simulink library "powerlib_models"  (Simulink 6.0)
settings: Solver=ode45  SolverMode=SingleTasking  StartTime=0.0  StopTime=10.0  RelTol=1e-3
values from neighbouring files (symbols this model uses):
  Ts = get(handles.edit1,'string')    [powergui.m]
undefined symbols (not defined in the file or in its folder): A, a0, a1, a2, a3, a4, a5, Ac, Amplitude, Amplitudes, B, BaseCurrent, BaseFlux, Bc, C, Capacitance, Cc, Columns, ConnectionType, Cs, ctrl, current, Current, damp, Dc, Dd, DiscIntNeverNeededParam, dref, dwo, exc, excAxis, F, Flux, fnom, Frequency, FreqVps, Gain1, gate, GH, GHd, GI, GId, GL, GLd, H, HarmonicGeneration, HT, hyd, I1_init, ib, ib2, Id1o, Inductance, InitialFlux, InitialSlope, io, Iq1o, isfinite, j, J ... (+138)
libraries: powerlib_models x32, powerlib_extras x4
(part 2 of 11)

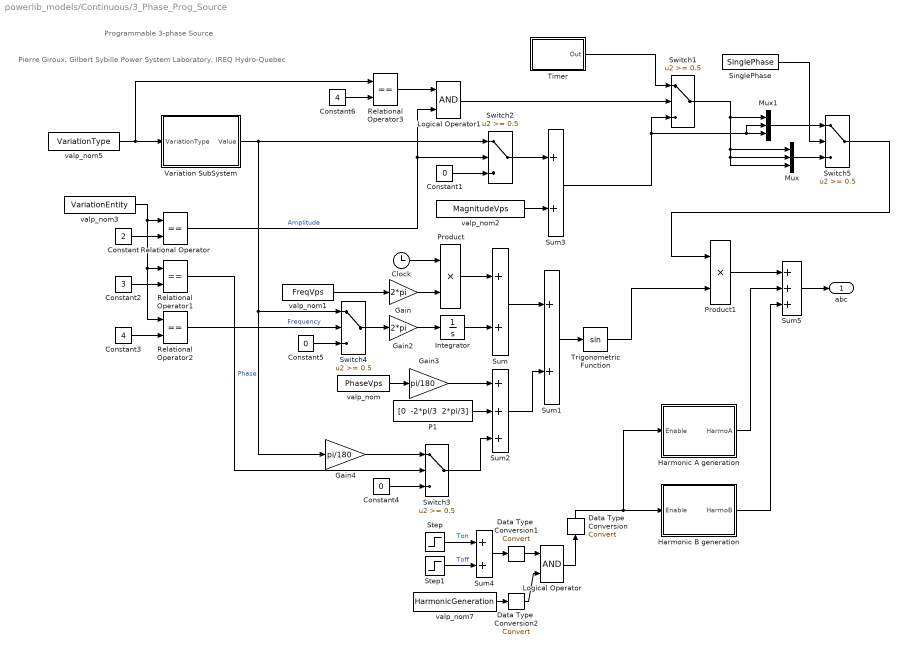
== system powerlib_models/Continuous/3_Phase_Prog_Source ==
  note: Pierre Giroux, Gilbert Sybille
      | Power System Laboratory, IREQ
      | Hydro-Quebec
  note: Programmable 3-phase Source
  Clock : Clock
  Constant : Constant  Value=2
  Constant1 : Constant  Value=0
  Constant2 : Constant  Value=3
  Constant3 : Constant  Value=4
  Constant4 : Constant  Value=0
  Constant5 : Constant  Value=0
  Constant6 : Constant  Value=4
  Data Type  Conversion : DataTypeConversion  Orientation=up  OutDataTypeMode=double  SaturateOnIntegerOverflow=on  RndMeth=Zero
  Data Type  Conversion1 : DataTypeConversion  OutDataTypeMode=boolean  SaturateOnIntegerOverflow=on  RndMeth=Zero
  Data Type  Conversion2 : DataTypeConversion  OutDataTypeMode=boolean  SaturateOnIntegerOverflow=on  RndMeth=Zero
  Gain : Gain  Gain=2*pi  SaturateOnIntegerOverflow=on
  Gain2 : Gain  Gain=2*pi  SaturateOnIntegerOverflow=on
  Gain3 : Gain  Gain=pi/180  SaturateOnIntegerOverflow=on
  Gain4 : Gain  Gain=pi/180  SaturateOnIntegerOverflow=on
  Harmonic A generation : Subsystem  mask(Harmonic generation){Freq_Vps=FreqVps, n_Harmo=n_HarmoA, Mag_Harmo=Mag_HarmoA, Phase_Harmo=Phase_HarmoA, Seq_Harmo=Seq_HarmoA, Ts=0}
      mask prompts: Ts "Sample time:"
  Harmonic B generation : Subsystem  mask(Harmonic generation){Freq_Vps=FreqVps, n_Harmo=n_HarmoB, Mag_Harmo=Mag_HarmoB, Phase_Harmo=Phase_HarmoB, Seq_Harmo=Seq_HarmoB, Ts=0}
      mask prompts: Ts "Sample time:"
  Integrator : Integrator
  Logical Operator : Logic
  Logical Operator1 : Logic
  Mux : Mux  Inputs=3
  Mux1 : Mux  Inputs=3
  P1 : Constant  Value="[0  -2*pi/3  2*pi/3]"
  Product : Product  SaturateOnIntegerOverflow=on  InputSameDT=on
  Product1 : Product  SaturateOnIntegerOverflow=on  InputSameDT=on
  Relational Operator{,1..3} (4 alike) : RelationalOperator  Operator===  InputSameDT=on
  SinglePhase : Constant  Value=SinglePhase
  Step : Step  Time=Ton_Harmo  SampleTime=0
  Step1 : Step  Time=Toff_Harmo  After=-1  SampleTime=0
  Sum{,1,3..4} (4 alike) : Sum  SaturateOnIntegerOverflow=on  InputSameDT=on
  Sum2 : Sum  Inputs=+++  SaturateOnIntegerOverflow=on  InputSameDT=on
  Sum5 : Sum  Inputs=+++  SaturateOnIntegerOverflow=on  InputSameDT=on
  Switch{1..5} (5 alike) : Switch  Threshold=0.5  InputSameDT=on
  Timer : Subsystem  mask(Timer){t=TimeValues, e=Amplitudes, Ts=0}
      mask prompts: t "Time (s):"; e "Amplitude:"; Ts "Sample time (s)"
      mask help:
      | Generates a signal changing  at specified times.
      |
      | Value of the signal at time zero must  be specified.
      mask init:
      | tt=t;sv=e;
      | tv=[-1,tt(1),reshape(repmat(reshape(tt(2:end),1,length(tt)-1),2,1),1,2*length(tt)-2),tt(end)+1];
      | %sv=(sv(:)'~=0);
      | opv=[sv(1),reshape(repmat(sv(1:end-1),2,1),1,2*length(sv)-2),sv(end),sv(end)];
      mask Display: plot( tv(2:end-1), opv(2:end-1) )
  Trigonometric Function : Trigonometry
  Variation SubSystem : Subsystem  mask(Variation Subsystem){VariationStep=VariationStep, VariationRate=VariationRate, VariationFreq=VariationFrequency, VariationMag=VariationMagnitude, Ton_Variation=Ton_Variation, Toff_Variation=Toff_Variation, Ts=0}
      mask prompts: Ts "Sample time:"
  valp_nom : Constant  Value=PhaseVps
  valp_nom1 : Constant  Value=FreqVps
  valp_nom2 : Constant  Value=MagnitudeVps
  valp_nom3 : Constant  Value=VariationEntity
  valp_nom5 : Constant  Value=VariationType
  valp_nom7 : Constant  Value=HarmonicGeneration
  abc : Outport  InitialOutput=0
  wires:
  Logical Operator1/1 -> Switch1/2
  Relational Operator3/1 -> Logical Operator1/1
  Switch5/1 -> Product1/1
  Switch1/1 -> Mux1/1, Mux/3, Mux/2, Mux/1
  Mux/1 -> Switch5/3
  SinglePhase/1 -> Switch5/2
  Mux1/1 -> Switch5/1
  Timer/1(Out) -> Switch1/1
  Sum3/1 -> Mux1/2, Mux1/3, Switch1/3
  Constant6/1 -> Relational Operator3/2
  Gain4/1 -> Switch3/1
  Harmonic B generation/1(HarmoB) -> Sum5/3
  Step1/1 -> Sum4/2  "Toff"
  Step/1 -> Sum4/1  "Ton"
  Sum5/1 -> abc/1
  Harmonic A generation/1(HarmoA) -> Sum5/2
  Constant5/1 -> Switch4/3
  Constant3/1 -> Relational Operator2/2
  Constant2/1 -> Relational Operator1/2
  valp_nom3/1 -> Relational Operator1/1, Relational Operator2/1, Relational Operator/1
  Constant/1 -> Relational Operator/2
  Relational Operator2/1 -> Switch4/2  "Frequency"
  Switch4/1 -> Gain2/1
  Variation SubSystem/1(Value) -> Gain4/1, Switch4/1, Switch2/1
  Relational Operator1/1 -> Switch3/2  "Phase"
  Constant4/1 -> Switch3/3
  Switch3/1 -> Sum2/3
  valp_nom5/1 -> Relational Operator3/1, Variation SubSystem/1(VariationType)
  Relational Operator/1 -> Logical Operator1/2, Switch2/2  "Amplitude"
  valp_nom2/1 -> Sum3/2
  Sum2/1 -> Sum1/2
  Constant1/1 -> Switch2/3
  Switch2/1 -> Sum3/1
  Product1/1 -> Sum5/1
  valp_nom1/1 -> Gain/1
  valp_nom/1 -> Gain3/1
  Gain3/1 -> Sum2/1
  Trigonometric Function/1 -> Product1/2
  P1/1 -> Sum2/2
  Integrator/1 -> Sum/2
  Gain2/1 -> Integrator/1
  Sum1/1 -> Trigonometric Function/1
  Sum/1 -> Sum1/1
  Clock/1 -> Product/1
  Gain/1 -> Product/2
  Product/1 -> Sum/1
  Logical Operator/1 -> Data Type  Conversion/1
  Data Type  Conversion/1 -> Harmonic A generation/1(Enable), Harmonic B generation/1(Enable)
  Sum4/1 -> Data Type  Conversion1/1
  Data Type  Conversion1/1 -> Logical Operator/1
  valp_nom7/1 -> Data Type  Conversion2/1
  Data Type  Conversion2/1 -> Logical Operator/2

== system powerlib_models/Continuous/ASM_mechanics ==
  Tm : Inport  Port=1  LatchInput=off
  Te : Inport  Port=2  LatchInput=off
  1\p : Gain  Gain=1/p  SaturateOnIntegerOverflow=on
  1_2H : Gain  Gain=1/(2*H)  SaturateOnIntegerOverflow=on
  1_Tb2 : Gain  Gain=1/Tb2  SaturateOnIntegerOverflow=on
  F : Gain  Orientation=left  Gain=F  SaturateOnIntegerOverflow=on
  Gain : Gain  Gain=[Nb2;Tb2;1]  SaturateOnIntegerOverflow=on
  Integrator : Integrator  InitialCondition=wmo
  Integrator1 : Integrator  InitialCondition=tho
  Mux3 : Mux  Inputs=2
  Mux4 : Mux  Inputs=3
  Sum : Sum  Inputs=-+-  SaturateOnIntegerOverflow=on  InputSameDT=on
  web_psb : Gain  Gain=web_psb  SaturateOnIntegerOverflow=on
  m : Outport
  thr,wr : Outport  Port=2
  wires:
  Mux4/1 -> Gain/1  "w,Te,thr"
  Mux3/1 -> thr,wr/1
  Tm/1 -> 1_Tb2/1
  Sum/1 -> 1_2H/1
  1_2H/1 -> Integrator/1
  Integrator/1 -> F/1, Mux3/2, Mux4/1, web_psb/1
  F/1 -> Sum/3
  1_Tb2/1 -> Sum/1
  Te/1 -> Mux4/2, Sum/2
  web_psb/1 -> Integrator1/1
  1\p/1 -> Mux4/3
  Integrator1/1 -> 1\p/1, Mux3/1
  Gain/1 -> m/1

== system powerlib_models/Continuous/Dynamic_Load ==
  v : Inport  Port=1  LatchInput=off
  PQ : Inport  Port=2  LatchInput=off
  3-phase PLL1 : Subsystem  mask(3-phase PLL){Par_Init=[Pha_V0  fnom], ParK=[60 1400]}
      mask prompts: Par_Init "Initial inputs:[ Phase(degrees)   Frequency(Hz) ]"; ParK "Regulator gains [ Kp  Ki ]"
      mask help:
      | This Phase Locked Loop (PLL) system can be used  to synchronize on a set of variable frequency, three-phase sinusoidal signals.
      |
      | Input 1: Vector containing the normalized
      |              three-phase signals [Va Vb Vc]
      | Output 1:  Measured frequency (Hz) = w/(2pi)
      | Output 2:  Ramp w.t   varying between  0 and 2*pi,
      | synchronized on zero crossings of the fundamental (positive-sequence) of phase A.
      | Output 3: Vector [sin(wt) cos(wt)]
      mask init:
      | Kp=ParK(1);
      | Ki=ParK(2);
      | Phase_Init=Par_Init(1);
      | Finit=Par_Init(2);
  Break  Alg. Loop : Subsystem  Orientation=left
  Complex to Real-Imag : ComplexToRealImag  Orientation=left
  Demux : Demux  Outputs=2
  Ground : Ground  Orientation=left
  Mux1 : Mux  Orientation=left  Inputs=3
  Positive Sequence  current : Subsystem
  Real-Imag to Complex : RealImagToComplex
  Real-Imag to Complex1 : RealImagToComplex
  Selector : Selector  Orientation=left  Elements=1:2  InputPortWidth=3
  V> pu : Gain  Gain=1/Vbase  SaturateOnIntegerOverflow=on
  Variable Frequency Mean value1 : Subsystem  mask(Variable-Frequency Mean Value){Finit=fnom, Vinit=Mag_V0}
      mask prompts: Finit "Initial frequency (Hz):"; Vinit "Initial input (DC component):"
      mask help:
      | This  block computes the mean value of the input signal (port In) over a running window of one cycle of a specified frequency (port Freq).
      |
      | For the first cycle of simulation (specified by the parameter "Initial frequency"), the ouput is held to the value of the  "Initial input" parameter.
  Variable Frequency Mean value2 : Subsystem  mask(Variable-Frequency Mean Value){Finit=fnom, Vinit=0}
      mask prompts: Finit "Initial frequency (Hz):"; Vinit "Initial input (DC component):"
      mask help:
      | This  block computes the mean value of the input signal (port In) over a running window of one cycle of a specified frequency (port Freq).
      |
      | For the first cycle of simulation (specified by the parameter "Initial frequency"), the ouput is held to the value of the  "Initial input" parameter.
  dq0_to_abc Transformation : powerlib_extras/Measurements/dq0_to_abc Transformation  Orientation=left
  i : Outport  Orientation=left
  m : Outport  Port=2
  wires:
  Selector/1 -> i/1
  v/1 -> V> pu/1
  Break  Alg. Loop/1(Out) -> Complex to Real-Imag/1
  Positive Sequence  current/2(VPQ) -> m/1
  Real-Imag to Complex1/1 -> Positive Sequence  current/2(S_ext)
  Demux/2 -> Real-Imag to Complex1/2
  Demux/1 -> Real-Imag to Complex1/1
  PQ/1 -> Demux/1
  3-phase PLL1/1(Freq) -> Variable Frequency Mean value2/1(Freq), Variable Frequency Mean value1/1(Freq)
  3-phase PLL1/4(Sin_Cos) -> dq0_to_abc Transformation/2
  3-phase PLL1/2(Vd) -> Variable Frequency Mean value1/2(In)
  Complex to Real-Imag/2 -> Mux1/2
  Complex to Real-Imag/1 -> Mux1/1
  Positive Sequence  current/1(I1(A)) -> Break  Alg. Loop/1(In)
  dq0_to_abc Transformation/1 -> Selector/1
  Variable Frequency Mean value2/1(Mean) -> Real-Imag to Complex/2
  Variable Frequency Mean value1/1(Mean) -> Real-Imag to Complex/1
  Ground/1 -> Mux1/3
  3-phase PLL1/3(Vq) -> Variable Frequency Mean value2/2(In)
  Mux1/1 -> dq0_to_abc Transformation/1
  Real-Imag to Complex/1 -> Positive Sequence  current/1(V1(pu))
  V> pu/1 -> 3-phase PLL1/1(Vab_bc (pu))

== system powerlib_models/Continuous/Excitation_System ==
  vref : Inport  Port=1  LatchInput=off
  vd : Inport  Port=2  LatchInput=off
  vq : Inport  Port=3  LatchInput=off
  vstab : Inport  Port=4  LatchInput=off
  Damping kf.s | (tf.s+1) : Subsystem  Orientation=left  mask(Transfer Function with Initial Outputs){N=[kf 0], D=[ tf 1], Y0=0, U0=v0(2)}
      mask prompts: N "Numerator:"; D "Denominator:"; Y0 "Initial output:"; U0 "Initial input:"
      mask help: Vector expressions for numerator, and denominator. Coefficients are in descending powers of s.
      mask init:
      | [A,B,C,Dd]=tf2ss(N,D);if (isempty(Y0));[m,n]=size(A);X0=zeros(1,m); end; if (isempty(U0));[m,p]=size(B);U0=zeros(1,p);end;
      |  if isempty(A),  X0=[]; else ,X0=getxo(A,B,C,Dd,U0,Y0,0); end
      mask Help: Specify the initial output for the transfer function.  An optimization routine attempts to determine the appropriate initial states so that the specified initial output is achieved.  For more details, see the m-file getxo.m
      mask Display: dpoly(N,D,'s')
  Exciter 1| (te.s+ke) : Subsystem  mask(Transfer Function with Initial Outputs){N=1, D=[ te ke], Y0=v0(2), U0=ke*v0(2)}
      mask prompts: N "Numerator:"; D "Denominator:"; Y0 "Initial output:"; U0 "Initial input:"
      mask help: Vector expressions for numerator, and denominator. Coefficients are in descending powers of s.
      mask init:
      | [A,B,C,Dd]=tf2ss(N,D);if (isempty(Y0));[m,n]=size(A);X0=zeros(1,m); end; if (isempty(U0));[m,p]=size(B);U0=zeros(1,p);end;
      |  if isempty(A),  X0=[]; else ,X0=getxo(A,B,C,Dd,U0,Y0,0); end
      mask Help: Specify the initial output for the transfer function.  An optimization routine attempts to determine the appropriate initial states so that the specified initial output is achieved.  For more details, see the m-file getxo.m
      mask Display: dpoly(N,D,'s')
  Lead Lag Compensator (tc.s+1) | (tb.s+1) : Subsystem  mask(Transfer Function with Initial Outputs){N=[tc 1], D=[tb 1], Y0=ke*v0(2)/ka, U0=ke*v0(2)/ka}
      mask prompts: N "Numerator:"; D "Denominator:"; Y0 "Initial output:"; U0 "Initial input:"
      mask help: Vector expressions for numerator, and denominator. Coefficients are in descending powers of s.
      mask init:
      | [A,B,C,Dd]=tf2ss(N,D);if (isempty(Y0));[m,n]=size(A);X0=zeros(1,m); end; if (isempty(U0));[m,p]=size(B);U0=zeros(1,p);end;
      |  if isempty(A),  X0=[]; else ,X0=getxo(A,B,C,Dd,U0,Y0,0); end
      mask Help: Specify the initial output for the transfer function.  An optimization routine attempts to determine the appropriate initial states so that the specified initial output is achieved.  For more details, see the m-file getxo.m
      mask Display: dpoly(N,D,'s')
  Low Pass Filter 1 | (tr.s+1) : Subsystem  mask(Transfer Function with Initial Outputs){N=1, D=[ tr 1], Y0=v0(1), U0=v0(1)}
      mask prompts: N "Numerator:"; D "Denominator:"; Y0 "Initial output:"; U0 "Initial input:"
      mask help: Vector expressions for numerator, and denominator. Coefficients are in descending powers of s.
      mask init:
      | [A,B,C,Dd]=tf2ss(N,D);if (isempty(Y0));[m,n]=size(A);X0=zeros(1,m); end; if (isempty(U0));[m,p]=size(B);U0=zeros(1,p);end;
      |  if isempty(A),  X0=[]; else ,X0=getxo(A,B,C,Dd,U0,Y0,0); end
      mask Help: Specify the initial output for the transfer function.  An optimization routine attempts to determine the appropriate initial states so that the specified initial output is achieved.  For more details, see the m-file getxo.m
      mask Display: dpoly(N,D,'s')
  Main Regulator ka | (ta.s +1) : Subsystem  mask(Transfer Function with Initial Outputs){N=ka, D=[ ta 1], Y0=ke*v0(2), U0=ke*v0(2)/ka}
      mask prompts: N "Numerator:"; D "Denominator:"; Y0 "Initial output:"; U0 "Initial input:"
      mask help: Vector expressions for numerator, and denominator. Coefficients are in descending powers of s.
      mask init:
      | [A,B,C,Dd]=tf2ss(N,D);if (isempty(Y0));[m,n]=size(A);X0=zeros(1,m); end; if (isempty(U0));[m,p]=size(B);U0=zeros(1,p);end;
      |  if isempty(A),  X0=[]; else ,X0=getxo(A,B,C,Dd,U0,Y0,0); end
      mask Help: Specify the initial output for the transfer function.  An optimization routine attempts to determine the appropriate initial states so that the specified initial output is achieved.  For more details, see the m-file getxo.m
      mask Display: dpoly(N,D,'s')
  Mux : Mux  Inputs=2
  Positive Sequence Voltage : Fcn  Expr=sqrt(u(1)^2 + u(2)^2)
  Proportionnal Saturation : Subsystem
  Sum : Sum  Inputs=++-+-  SaturateOnIntegerOverflow=on  InputSameDT=on
  Vf0| ka : Constant  Value=v0(2)/ka
  Vf : Outport  InitialOutput=0
  wires:
  Proportionnal Saturation/1(Ef) -> Exciter 1| (te.s+ke)/1(In1)
  Lead Lag Compensator (tc.s+1) | (tb.s+1)/1(Out1) -> Main Regulator ka | (ta.s +1)/1(In1)
  Sum/1 -> Lead Lag Compensator (tc.s+1) | (tb.s+1)/1(In1)
  Positive Sequence Voltage/1 -> Low Pass Filter 1 | (tr.s+1)/1(In1)
  vq/1 -> Mux/2
  vd/1 -> Mux/1
  Mux/1 -> Positive Sequence Voltage/1
  vref/1 -> Sum/1
  vstab/1 -> Sum/4
  Low Pass Filter 1 | (tr.s+1)/1(Out1) -> Proportionnal Saturation/2(Vtf), Sum/3
  Vf0| ka/1 -> Sum/2
  Main Regulator ka | (ta.s +1)/1(Out1) -> Proportionnal Saturation/1(Efd)
  Damping kf.s | (tf.s+1)/1(Out1) -> Sum/5
  Exciter 1| (te.s+ke)/1(Out1) -> Damping kf.s | (tf.s+1)/1(In1), Vf/1

== system powerlib_models/Continuous/GTO-IGBT Bridge ==
  note: GTO:
      |  tail current can be turned off by specifying Tf=0 and Tt=0
  note: Diode Logic :
      | 1) Diodes are blocked when complementary GTOs are switched on
      | 2) When no snubber capacitances are used (Cs=inf), diodes are triggered
      | when complementary GTOs are swithed off
  note: 6
  note: 5
  note: ***********************************************
  note: C
  note: *
      | *
      | ||
      | ||
      | *
      | *
      | *
      | ||
      | ||
      | *
      | *
  note: B
  note: A
  note: Vcc
  note: ***********************************************
  note: 4
  note: 3
  note: *
      | *
      | ||
      | ||
      | *
      | *
      | *
      | ||
      | ||
      | *
      | *
  note: -
  note: +
  note: 2
  note: 1
  note: *
      | *
      | ||
      | ||
      | *
      | *
      | *
      | ||
      | ||
      | *
      | *
  "v " : Inport  Port=1  LatchInput=off
  g : Inport  Port=2  LatchInput=off
  1/Rsw : Gain  Orientation=up  Gain=1./Rsw  SaturateOnIntegerOverflow=on
  2 : Constant  Value=Tf>0 | Tt>0
  Constant1 : Constant  Value=0
  Data Type  Conversion1 : DataTypeConversion  OutDataTypeMode=double  SaturateOnIntegerOverflow=on  RndMeth=Zero
  Data Type  Conversion3 : DataTypeConversion  OutDataTypeMode=double  SaturateOnIntegerOverflow=on  RndMeth=Zero
  Data Type  Conversion4 : DataTypeConversion  OutDataTypeMode=boolean  SaturateOnIntegerOverflow=on  RndMeth=Zero
  Data Type  Conversion5 : DataTypeConversion  OutDataTypeMode=boolean  SaturateOnIntegerOverflow=on  RndMeth=Zero
  Diode Logic : Subsystem
  GTO Logic : Subsystem
  G_D : Logic  Operator=OR
  Gain : Gain  Orientation=up  Gain=-1  SaturateOnIntegerOverflow=on
  Memory : Memory  InheritSampleTime=on
  Memory1 : Memory  InheritSampleTime=on
  Memory2 : Memory  InheritSampleTime=on
  Product : Product  SaturateOnIntegerOverflow=on  InputSameDT=on
  Relational Operator : RelationalOperator  InputSameDT=on
  "Tail " : Subsystem  TreatAsAtomicUnit=on  mask(Gto tail current){Tf=Tf, Tt=Tt}
      mask prompts: Tf "Current 10% fall time Tf (s) :"; Tt "Current tail time Tt (s) :"
  "Vf " : Subsystem
  iTail : Outport
  Status : Outport  Port=2
  Vf : Outport  Port=3
  wires:
  Memory2/1 -> Vf/1
  GTO Logic/1(status) -> "Vf "/1(status_GTO), Diode Logic/3(G), G_D/2
  "Vf "/1(Vf) -> Memory2/1
  "v "/1 -> Gain/1, GTO Logic/1(Vak), 1/Rsw/1
  "Tail "/1(itail) -> iTail/1
  2/1 -> "Tail "/Enable
  G_D/1 -> Memory/1
  Constant1/1 -> Relational Operator/2
  Memory1/1 -> "Tail "/1(Iak)
  Gain/1 -> Diode Logic/1(Vak)
  Product/1 -> Memory1/1  "IGTO"
  Memory/1 -> Data Type  Conversion1/1
  Data Type  Conversion1/1 -> Status/1
  Data Type  Conversion3/1 -> Product/1
  Relational Operator/1 -> Data Type  Conversion3/1, Diode Logic/2(Ipos)
  g/1 -> Data Type  Conversion4/1
  Data Type  Conversion4/1 -> "Tail "/2(switch), GTO Logic/2(G)
  Diode Logic/1(status) -> Data Type  Conversion5/1
  Data Type  Conversion5/1 -> G_D/1
  1/Rsw/1 -> Relational Operator/1, Product/2

== system powerlib_models/Continuous/HTG ==
  wref : Inport  Port=1  LatchInput=off
  Pref : Inport  Port=2  LatchInput=off
  we : Inport  Port=3  LatchInput=off
  Pe : Inport  Port=4  LatchInput=off
  dw : Inport  Port=5  LatchInput=off
  Constant1 : Constant  Orientation=left  Value=dref
  PID : Subsystem
      mask Type: PID(2) Controller
      mask Display: disp('PID')
  Sum : Sum  Inputs=+-  SaturateOnIntegerOverflow=on  InputSameDT=on
  Sum1 : Sum  Inputs=+-  SaturateOnIntegerOverflow=on  InputSameDT=on
  Sum5 : Sum  Inputs=-+  SaturateOnIntegerOverflow=on  InputSameDT=on
  Switch : Switch  Orientation=left  Threshold=0.5  InputSameDT=on
  permanent droop : Gain  Orientation=left  Gain=Rp  SaturateOnIntegerOverflow=on
  servo-motor : Subsystem
      mask Display: disp('servo-\nmotor')
  turbine : Subsystem
      mask Display: disp('hydraulic\nturbine')
  Pm : Outport  InitialOutput=0
  gate : Outport  Port=2  InitialOutput=0
  wires:
  Constant1/1 -> Switch/2
  Switch/1 -> permanent droop/1
  Pe/1 -> Sum5/2
  Pref/1 -> Sum5/1
  Sum1/1 -> PID/1(error)
  permanent droop/1 -> Sum1/2
  Sum/1 -> Sum1/1
  PID/1(Output) -> servo-motor/1(regulator's output)
  wref/1 -> Sum/1
  we/1 -> Sum/2
  Sum5/1 -> Switch/3
  servo-motor/1(gate opening) -> turbine/2(gate opening), gate/1, Switch/1
  dw/1 -> turbine/1(dw)
  turbine/1(Pm) -> Pm/1

== system powerlib_models/Continuous/Impedance Measurement ==
  v : Inport  Port=1  LatchInput=off
  Ground : Ground
  Terminator : Terminator
  i : Outport  InitialOutput=0
  wires:
  Ground/1 -> i/1
  v/1 -> Terminator/1

== system powerlib_models/Continuous/MBPSS ==
  note: Innocent Kamwa, Robert Grondin
      | IREQ, Hydro-Quebec
  note: Multi-band Power System Stabilizer
  note: (IEEE Type PSS4b)
  note: Note: Speed deviation is derived from the machine positive-sequence terminal voltages and currents.
  note: Low and intermediate speed deviation is based on the internal voltage phasors while
      | the high frequency speed deviation  is based on the electrical power.
  note: (for simplified
      | settings only)
  dw : Inport  Port=1  LatchInput=off
  BF1 : TransferFcn  Numerator=[TL1 KL11]  Denominator=[TL2 1]
  BF7 : TransferFcn  Numerator=[TL7 KL17]  Denominator=[TL8 1]
  Constant : Constant  Value=Detailed
  Gain : Gain  Gain=KL  SaturateOnIntegerOverflow=on
  Gain1 : Gain  Gain=KI  SaturateOnIntegerOverflow=on
  Gain2 : Gain  Gain=KH  SaturateOnIntegerOverflow=on
  Gain3 : Gain  Gain=KL1  SaturateOnIntegerOverflow=on
  Gain4 : Gain  Gain=KL2  SaturateOnIntegerOverflow=on
  Gain5 : Gain  Gain=KI1  SaturateOnIntegerOverflow=on
  Gain6 : Gain  Gain=KI2  SaturateOnIntegerOverflow=on
  Gain7 : Gain  Gain=KH1  SaturateOnIntegerOverflow=on
  Gain8 : Gain  Gain=KH2  SaturateOnIntegerOverflow=on
  Gain9 : Gain  Gain=Kg  SaturateOnIntegerOverflow=on
  HF speed sensor : TransferFcn  Numerator="[80  0 0]"  Denominator=[1 82 161 80]
  HF1 : TransferFcn  Numerator=[TH1 KH11]  Denominator=[TH2 1]
  HF4 : TransferFcn  Numerator=[TH7 KH17]  Denominator=[TH8 1]
  IF1 : TransferFcn  Numerator=[TI1 KI11]  Denominator=[TI2 1]
  IF4 : TransferFcn  Numerator=[TI7 KI17]  Denominator=[TI8 1]
  LF and IF speed sensor : TransferFcn  Numerator=[-1.759e-3 1]  Denominator=[1.2739e-4 1.7823e-2 1]
  "Limiteur BF " : Saturate  UpperLimit=LIM_VL  LowerLimit=-LIM_VL
  Limiteur HF : Saturate  UpperLimit=LIM_VH  LowerLimit=-LIM_VH
  "Limiteur IF " : Saturate  UpperLimit=LIM_VI  LowerLimit=-LIM_VI
  Limiteur VS : Saturate  UpperLimit=LIM_VS  LowerLimit=-LIM_VS
  Sum : Sum  Inputs=+-  SaturateOnIntegerOverflow=on  InputSameDT=on
  Sum1 : Sum  Inputs=+++  SaturateOnIntegerOverflow=on  InputSameDT=on
  Sum2 : Sum  Inputs=+-  SaturateOnIntegerOverflow=on  InputSameDT=on
  Sum3 : Sum  Inputs=+-  SaturateOnIntegerOverflow=on  InputSameDT=on
  Transfer function for detailed model (HF) : Subsystem
  Transfer function for detailed model (IF) : Subsystem
  Transfer function for detailed model (LF) : Subsystem
  VS : Outport  InitialOutput=0
  wires:
  dw/1 -> LF and IF speed sensor/1, HF speed sensor/1
  HF speed sensor/1 -> Gain7/1, Gain8/1
  LF and IF speed sensor/1 -> Gain6/1, Gain5/1, Gain4/1, Gain3/1
  Gain8/1 -> HF4/1
  Gain7/1 -> HF1/1
  Gain6/1 -> IF4/1
  Gain5/1 -> IF1/1
  Gain4/1 -> BF7/1
  Gain3/1 -> BF1/1
  Gain2/1 -> Limiteur HF/1
  Gain1/1 -> "Limiteur IF "/1
  Gain/1 -> "Limiteur BF "/1
  Sum/1 -> Gain/1
  Transfer function for detailed model (LF)/1(LFpos) -> Sum/1
  Transfer function for detailed model (LF)/2(LFneg) -> Sum/2
  BF1/1 -> Transfer function for detailed model (LF)/2("LFpos ")
  BF7/1 -> Transfer function for detailed model (LF)/3("LFneg ")
  Transfer function for detailed model (IF)/1(IFpos) -> Sum2/1
  Transfer function for detailed model (IF)/2(LFneg) -> Sum2/2
  IF1/1 -> Transfer function for detailed model (IF)/2("IFpos ")
  IF4/1 -> Transfer function for detailed model (IF)/3("IFneg ")
  Sum2/1 -> Gain1/1
  HF1/1 -> Transfer function for detailed model (HF)/2("HFpos ")
  HF4/1 -> Transfer function for detailed model (HF)/3("HFneg ")
  Transfer function for detailed model (HF)/1(HFpos) -> Sum3/1
  Transfer function for detailed model (HF)/2(HFneg) -> Sum3/2
  Sum3/1 -> Gain2/1
  "Limiteur BF "/1 -> Sum1/1
  "Limiteur IF "/1 -> Sum1/2
  Limiteur HF/1 -> Sum1/3
  Sum1/1 -> Gain9/1
  Limiteur VS/1 -> VS/1
  Constant/1 -> Transfer function for detailed model (LF)/1(On), Transfer function for detailed model (IF)/1(On), Transfer function for detailed model (HF)/1(On)
  Gain9/1 -> Limiteur VS/1

== system powerlib_models/Continuous/Measurement ==
  note: The Measurement is not modified
  in : Inport  Port=1  LatchInput=off
  out : Outport
  wires:
  in/1 -> out/1

== system powerlib_models/Continuous/PMSM_mechanics ==
  Tm : Inport  Port=1  LatchInput=off
  Te : Inport  Port=2  LatchInput=off
  Gain : Gain  Gain=p  SaturateOnIntegerOverflow=on
  Gain1 : Gain  Gain=1/p  SaturateOnIntegerOverflow=on
  Gain2 : Gain  Gain=1/J  SaturateOnIntegerOverflow=on
  Gain3 : Gain  Gain=F  SaturateOnIntegerOverflow=on
  Int : Integrator
  Int1 : Integrator
  Mux1 : Mux  Inputs=3
  Sum : Sum  Inputs=-+-  SaturateOnIntegerOverflow=on  InputSameDT=on
  we : Outport  InitialOutput=0
  the : Outport  Port=2  InitialOutput=0
  m : Outport  Port=3  InitialOutput=0
  wires:
  Int1/1 -> Gain1/1, the/1
  Gain1/1 -> Mux1/2
  Te/1 -> Mux1/3, Sum/2
  Gain/1 -> we/1, Int1/1
  Int/1 -> Mux1/1, Gain3/1, Gain/1
  Gain2/1 -> Int/1
  Sum/1 -> Gain2/1
  Tm/1 -> Sum/1
  Mux1/1 -> m/1
  Gain3/1 -> Sum/3

== system powerlib_models/Continuous/PM_synchronous_machine ==
  v : Inport  Port=1  LatchInput=off
  we : Inport  Port=2  LatchInput=off
  the : Inport  Port=3  LatchInput=off
  Mux : Mux  Inputs=[3,2,2]
  Selector : Selector  Elements=1:2  InputPortWidth=3
  "Te " : Fcn  Expr=1.5*p*(Flux*u(1)+(Ld-Lq)*u(1)*u(2))
  abc2qd : Subsystem
  iq,id : Subsystem
  qd2abc : Subsystem
  i : Outport  InitialOutput=0
  m : Outport  Port=2  InitialOutput=0
  Te : Outport  Port=3  InitialOutput=0
  wires:
  Selector/1 -> i/1
  qd2abc/1(is) -> Selector/1, Mux/1  "isabc"
  iq,id/1(iq,id) -> qd2abc/2(iq,id), "Te "/1, Mux/2  "iqd"
  v/1 -> abc2qd/1(Vab,Vbc)
  abc2qd/1(s,c) -> qd2abc/1(s,c)
  abc2qd/2(vq,vd) -> iq,id/1(vq,vd), Mux/3  "vqd"
  Mux/1 -> m/1
  we/1 -> iq,id/2(we)
  the/1 -> abc2qd/2(the)
  "Te "/1 -> Te/1

== system powerlib_models/Continuous/PSS ==
  note: Power System Stabilizer (PSS)
      | (generic model)
  In : Inport  Port=1  LatchInput=off
  Lead-lag #1 : TransferFcn  Numerator=[T1n 1]  Denominator=[T1d 1]
  Lead-lag #2 : TransferFcn  Numerator=[T2n 1]  Denominator=[T2d 1]
  "Limiter " : Saturate  UpperLimit=VSlimits(2)  LowerLimit=VSlimits(1)
  Overall Gain : Gain  Gain=K  SaturateOnIntegerOverflow=on
  Sensor : Subsystem  AncestorBlock=|  mask(Discrete 1st-Order Filter){FilterType=Lowpass, Tc=Tsensor, Initialize=on, Vac_Init=[0 0 60], Vdc_Init=Vinit, PlotResponse=off, param1=[1 500 1]}
      | powerlib_extras/Control 
      | Blocks/1st-Order 
      | Filter
      mask prompts: FilterType "Filter Type:"; Tc "Time constant (s):"; Initialize "Initialize filter states"; Vac_Init "AC initial input: [ Mag  Phase(degrees)  Freq(Hz) ]"; Vdc_Init "DC Initial input:"; PlotResponse "Plot filter response"; param1 "Frequency range(Hz) : [Start  End  Inc.]"
      mask init:
      | switch FilterType
      | case 1, % Lowpass
      |        X=[0 1 2 3 4];
      |        Y=[-2 -2 -3 -4 -4];
      |        numc=1;
      |        denc=[Tc 1];
      |  case 2,   % Highpass
      |        X=[0 1 2 3 4];
      |        Y=[-4 -4 -3 -2 -2];
      |         numc=[1 0];
      |         denc=[1 1/Tc];
      | end
      | %
      | [Ac,Bc,Cc,Dc]=tf2ss(numc,denc);
      | %
      | %
      | if Initialize==1  % Compute initial conditions on states
      | u1=Vac_Init(1)*exp(j*Vac_Init(2)*pi/180);
      | u2=Vdc_Init*exp(j*90*pi/180);
      | u=u1+u2;
      | u0=imag(u); % input at  t=0;
      | I=eye(size(Ac));
      | sI1=I*j*(2*pi*Vac_Init(3));
      | sI2=I*j*0;
      | x=inv(sI1-Ac)*Bc*u1 + inv(sI2-Ac)*Bc*u2;
      | x0c=imag(x);
      | else
      | x0c=0;
      | end
      | %
      | if PlotResponse==1 % Plot frequency and step response
      | figure(1)
      | sys=ss(Ac,Bc,Cc,Dc);
      | f=param1(1):param1(3):param1(2);
      | w=2*pi*f;
      | [mag phase]=bode(sys,w);
      | subplot(2,1,1)
      | plot(f,squeeze(mag))
      | title('Magnitude')
      | grid
      | subplot(2,1,2)
      | plot(f,squeeze(phase))
      | title('Phase (degrees)')
      | xlabel('Hz')
      | grid
      | figure(2)
      | step(sys)
      | end
      mask StyleString: popup(Lowpass|Highpass),edit,checkbox,edit,edit,checkbox,edit
      mask CallbackString: ||parametres=get_param(gcb,'MaskValues');p3=parametres{3};p6=parametres{6};if strcmp(p3,'on');param4='on';param5='on';else;param4='off';param5='off';end;if strcmp(p6,'on');param7='on';else;param7='off';end;visible={'on','on','on',param4,param5,'on',param7};set_param(gcb,'MaskVisibilities',visible)|||parametres=get_param(gcb,'MaskValues');p3=parametres{3};p6=parametres{6};if strcmp(p3,'on');param4='on';param5='on';else;param4='off';param5='off';end;if strcmp(p6,'on');param7='on';else;param7='off';end;visible={'on','on','on',param4,param5,'on',param7};set_param(gcb,'MaskVisibilities',visible)|
      mask Display: plot(X,Y);
  Wash-out : Subsystem  AncestorBlock=|  mask(Discrete 1st-Order Filter){FilterType=Highpass, Tc=Twashout, Initialize=on, Vac_Init=[0 0 60], Vdc_Init=K*Vinit, PlotResponse=off, param1=[1 500 1]}
      | powerlib_extras/Control 
      | Blocks/1st-Order 
      | Filter
      mask prompts: FilterType "Filter Type:"; Tc "Time constant (s):"; Initialize "Initialize filter states"; Vac_Init "AC initial input: [ Mag  Phase(degrees)  Freq(Hz) ]"; Vdc_Init "DC Initial input:"; PlotResponse "Plot filter response"; param1 "Frequency range(Hz) : [Start  End  Inc.]"
      mask init: same as powerlib_models/Continuous/PSS/Sensor
      mask StyleString: popup(Lowpass|Highpass),edit,checkbox,edit,edit,checkbox,edit
      mask CallbackString: ||parametres=get_param(gcb,'MaskValues');p3=parametres{3};p6=parametres{6};if strcmp(p3,'on');param4='on';param5='on';else;param4='off';param5='off';end;if strcmp(p6,'on');param7='on';else;param7='off';end;visible={'on','on','on',param4,param5,'on',param7};set_param(gcb,'MaskVisibilities',visible)|||parametres=get_param(gcb,'MaskValues');p3=parametres{3};p6=parametres{6};if strcmp(p3,'on');param4='on';param5='on';else;param4='off';param5='off';end;if strcmp(p6,'on');param7='on';else;param7='off';end;visible={'on','on','on',param4,param5,'on',param7};set_param(gcb,'MaskVisibilities',visible)|
      mask Display: plot(X,Y);
  VS : Outport  InitialOutput=0
  wires:
  "Limiter "/1 -> VS/1
  Lead-lag #2/1 -> "Limiter "/1
  Lead-lag #1/1 -> Lead-lag #2/1
  Wash-out/1(Out) -> Lead-lag #1/1
  Overall Gain/1 -> Wash-out/1(In)
  Sensor/1(Out) -> Overall Gain/1
  In/1 -> Sensor/1(In)

== system powerlib_models/Continuous/SM_mechanics ==
  note: This subsystem models the mechanical part of the synchronous machine.
  "Te " : Inport  Port=1  PortDimensions=1  LatchInput=off
  Pm : Inport  Port=2  PortDimensions=1  LatchInput=off
  1_(2H) : Gain  Gain=1/(2*H)  SaturateOnIntegerOverflow=on
  1_Pb : Gain  Gain=1/Pb  SaturateOnIntegerOverflow=on
  Clock : Clock
      settings: Decimation=10
  F1 : Gain  Orientation=left  Gain=F  SaturateOnIntegerOverflow=on
  Fcn1 : Fcn  Expr=rem(u,2*pi)
  Integrator : Integrator  InitialCondition=dwo
  Integrator1 : Integrator  InitialCondition=tho
  Integrator2 : Integrator  InitialCondition=tho
  Mux1 : Mux  Inputs=2
  Mux2 : Mux  Inputs=[1,1,1,1,1,1]
  Product : Product  SaturateOnIntegerOverflow=on  InputSameDT=on
  Sum : Sum  SaturateOnIntegerOverflow=on  InputSameDT=on
  Sum2 : Sum  Inputs=+--  SaturateOnIntegerOverflow=on  InputSameDT=on
  Sum3 : Sum  SaturateOnIntegerOverflow=on  InputSameDT=on
  div : Fcn  Expr=u[2]/u[1]
      mask Display: disp('/')
  nom. speed : Constant
  theta : Gain  Gain=180/pi  SaturateOnIntegerOverflow=on
  units : Gain  Gain=Nb  SaturateOnIntegerOverflow=on
  units1 : Gain  Gain=Pb  SaturateOnIntegerOverflow=on
  units2 : Gain  Gain=Pb/Nb  SaturateOnIntegerOverflow=on
  web1 : Gain  Gain=web_psb  SaturateOnIntegerOverflow=on
  web2 : Gain  Gain=web_psb  SaturateOnIntegerOverflow=on
  web3 : Gain  Gain=web_psb  SaturateOnIntegerOverflow=on
  m : Outport  InitialOutput=0
  theta_e : Outport  Port=2  InitialOutput=0
  we : Outport  Port=3  InitialOutput=0
  wires:
  units2/1 -> Mux2/6  "Te"
  units1/1 -> Mux2/3  "Pe"
  units/1 -> Mux2/2  "n"
  Mux2/1 -> m/1  "Mechanical"
  theta/1 -> Mux2/5  "theta"
  Fcn1/1 -> theta/1
  Integrator1/1 -> Fcn1/1  "d_theta (rad)"
  web3/1 -> Integrator1/1
  Sum3/1 -> theta_e/1
  Sum/1 -> F1/1, Product/1, units/1, web3/1, Mux1/1, we/1  "n"
  Sum2/1 -> 1_(2H)/1
  F1/1 -> Sum2/3
  1_Pb/1 -> Mux1/2
  Pm/1 -> 1_Pb/1
  Mux1/1 -> div/1
  "Te "/1 -> Sum2/2, Product/2, units2/1  "Te"
  div/1 -> Sum2/1
  1_(2H)/1 -> Integrator/1
  nom. speed/1 -> Sum/1
  Product/1 -> units1/1  "Pe"
  Integrator/1 -> Sum/2, web1/1, Mux2/4  "dw"
  web1/1 -> Integrator2/1
  Clock/1 -> web2/1
  web2/1 -> Sum3/2
  Integrator2/1 -> Mux2/1, Sum3/1  "d_theta (rad)"

== system powerlib_models/Continuous/SSM_mechanics ==
  Pm : Inport  Port=1  LatchInput=off
  Pe : Inport  Port=2  LatchInput=off
  1_(2*H) : Gain  Gain=1/(2*H)  SaturateOnIntegerOverflow=on
  1_Pb : Gain  Gain=1/Pb  SaturateOnIntegerOverflow=on
  Gain : Gain  Orientation=left  Gain=Kd  SaturateOnIntegerOverflow=on
  Integrator : Integrator  InitialCondition=dwo
  Integrator1 : Integrator  InitialCondition=tho
  Mux1 : Mux  Inputs=2
  Sum : Sum  SaturateOnIntegerOverflow=on  InputSameDT=on
  Sum1 : Sum  Inputs=+-  SaturateOnIntegerOverflow=on  InputSameDT=on
  Sum2 : Sum  Inputs=-+  SaturateOnIntegerOverflow=on  InputSameDT=on
  div : Fcn  Expr=u[2]/u[1]
      mask Display: disp('division')
  nom. speed : Constant
  web_psb : Gain  Gain=web_psb  SaturateOnIntegerOverflow=on
  theta_e : Outport  InitialOutput=0
  wm : Outport  Port=2  InitialOutput=0
  wires:
  nom. speed/1 -> Sum/1
  Integrator/1 -> Gain/1, Sum/2
  Sum1/1 -> 1_(2*H)/1
  Gain/1 -> Sum1/2
  div/1 -> Sum1/1
  1_(2*H)/1 -> Integrator/1
  Sum/1 -> web_psb/1, wm/1, Mux1/1
  Sum2/1 -> Mux1/2
  Pe/1 -> Sum2/1
  Mux1/1 -> div/1
  Integrator1/1 -> theta_e/1
  web_psb/1 -> Integrator1/1
  1_Pb/1 -> Sum2/2
  Pm/1 -> 1_Pb/1

== system powerlib_models/Continuous/Three-Level Bridge ==
  v : Inport  Port=1  PortDimensions=nb_arm*3  LatchInput=off
  g : Inport  Port=2  PortDimensions=nb_arm*4  LatchInput=off
  2-level GTO-IGBT Bridge  Logic (modified) : Subsystem  AncestorBlock=powerlib_models/Discrete/GTO-IGBT Bridge  mask(GTO & IGBT Bridge Logic(modified)){nb_arm=nb_arm, Tf=0, Tt=0, Cs=Cs, VFs=Par_Vf, Rsw=Ron, Ts=Ts}
      mask prompts: nb_arm "Number of bridge arms (1,2 or 3)"; Tf "Curent 10% fall time Tf (s) :"; Tt "Current tail time Tt (s) :"; Cs "Snubber Capacitance Cs (F):"; VFs "Forward Voltages [ Vf  Vfd ]"; Rsw "Device resistance"; Ts "Time step Ts (s) :"
      mask help:
      | Generates the switch status ( 0 or 1) and the tail currents for a forced-commutated two- level bridge using GTO/Diode or IGBT/Diode pairs.
      | Specify  3 arms (6 switches) for 3 phase bridge, 2 arms for 4 switches, or 1 arm.
      | To turn-off the tail current, specify Tf=0 and Tt=0.
      mask init:
      | Vf=VFs(1);
      | Vfd=VFs(2);
      | nb_switch=nb_arm*2;
      | if nb_arm==1,
      |    Selec_Diode=[2 1];
      |    Block3Elements=[1 2];
      |    VswElements=[1 2];
      | elseif nb_arm==2,
      |    Selec_Diode=[2 1 4 3];
      |    Block3Elements=[1 3 2 4];
      |    VswElements=[1 2 4 5];
      | elseif nb_arm==3,
      |    Selec_Diode=[2 1 4 3 6 5];
      |    Block3Elements=[1 3 5 2 4 6];
      |    VswElements=[1 2 4 5 7 8];
      | end
  Input : Subsystem
  Mux : Mux  Inputs=[nb_arm*2 nb_arm]
  Mux1 : Mux  Inputs=[nb_arm*2 nb_arm]
  Select_Status : Selector  Elements=StatusElements  InputPortWidth=3*nb_arm
  Select_Status1 : Selector  Elements=StatusElements  InputPortWidth=3*nb_arm
  SubSystem : Subsystem
      mask Display: disp('?')
  Sw3 (clamping diode) Logic : Subsystem  mask{nb_arm=nb_arm, VFs=Par_Vf, Ts=Ts}
      mask prompts: nb_arm "Number of bridge arm:"; VFs "Forward Voltages [ Vf  Vfd ]"; Ts "Sample time:"
      mask init:
      | Vf=VFs(1);
      | Vfd=VFs(2);
      | nb_switch=nb_arm*2;
      | if nb_arm==1,
      |    Vsw3Elements=[3];
      |    PulseElements=[1 2 3 4];
      |    g12Elements=[1 2];
      |   Trig12Elements=[1 2];
      | BlockDElements=[1 2];
      | elseif nb_arm==2,
      |    Vsw3Elements=[3 6];
      |    PulseElements=[1 5 2 6 3 7 4 8];
      |    g12Elements=[1 3 2 4];
      |   BlockDElements=[1 3 2 4];
      |   Trig12Elements=[1 3 2 4];
      | elseif nb_arm==3,
      |    Vsw3Elements=[3 6 9];
      |    PulseElements=[1 5 9 2 6 10 3 7 11 4 8 12];
      |    g12Elements=[1 4 2 5 3 6];
      |    BlockDElements=[1 4 2 5 3 6];
      |   Trig12Elements=[1 3 5 2 4 6];
      | end
  x : Outport
  Status : Outport  Port=2
  Vf : Outport  Port=3
  wires:
  2-level GTO-IGBT Bridge  Logic (modified)/4(status_GTO) -> Sw3 (clamping diode) Logic/4(Status_GTO)
  Input/1(Out) -> Sw3 (clamping diode) Logic/2(Pulses)
  g/1 -> Input/1(In)
  Sw3 (clamping diode) Logic/5(Trig12) -> 2-level GTO-IGBT Bridge  Logic (modified)/4(Trig12)
  v/1 -> 2-level GTO-IGBT Bridge  Logic (modified)/1(v), Sw3 (clamping diode) Logic/1(V_Sw123)
  2-level GTO-IGBT Bridge  Logic (modified)/1(status) -> Mux/1
  Mux1/1 -> Select_Status1/1
  Mux/1 -> Select_Status/1
  2-level GTO-IGBT Bridge  Logic (modified)/2(Vf) -> Mux1/1
  Sw3 (clamping diode) Logic/1(Status) -> Mux/2
  Sw3 (clamping diode) Logic/2(Vf) -> Mux1/2
  Sw3 (clamping diode) Logic/3(g12) -> 2-level GTO-IGBT Bridge  Logic (modified)/2(g)
  Sw3 (clamping diode) Logic/4(Block12) -> 2-level GTO-IGBT Bridge  Logic (modified)/3(Block12)
  2-level GTO-IGBT Bridge  Logic (modified)/3(Block3) -> Sw3 (clamping diode) Logic/3(Block3)
  Select_Status/1 -> Status/1
  Select_Status1/1 -> Vf/1, x/1

== system powerlib_models/Continuous/Xfohyst1Ph ==
  Goto2 : Terminator
  transformer : powerlib_models/Continuous/hysteresis_transformer  SaturationFlux=SaturationFlux  SaturationCurrent=SaturationCurrent  InitialFlux=InitialFlux1  FluxBase=BaseFlux  CurrentBase=BaseCurrent  Tolerances=Tolerances  HT=HT  UpperFlux=UpperFlux  LowerFlux=LowerFlux  Current=Current  InitialSlope=InitialSlope  TransfoNumber=TransfoNumber  sfun_InitialFlux=sfun_InitialFlux
  tag scope: LibraryTag=global
  wires:
  transformer/1 -> [LibraryTag]
  [LibraryTag] -> transformer/1
  transformer/2 -> Goto2/1

== system powerlib_models/Continuous/Xfohyst1PhF ==
  transformer : powerlib_models/Continuous/hysteresis_transformer  SaturationFlux=SaturationFlux  SaturationCurrent=SaturationCurrent  InitialFlux=InitialFlux  FluxBase=BaseFlux  CurrentBase=BaseCurrent  Tolerances=Tolerances  HT=HT  UpperFlux=UpperFlux  LowerFlux=LowerFlux  Current=Current  InitialSlope=InitialSlope  TransfoNumber=TransfoNumber  sfun_InitialFlux=sfun_InitialFlux
  tag scope: LibraryTag=global
  wires:
  [LibraryTag] -> transformer/1
  transformer/1 -> [LibraryTag]
  transformer/2 -> [LibraryTag]

== system powerlib_models/Continuous/Xfohyst3Ph ==
  Goto2 : Terminator
  Goto4 : Terminator
  Goto6 : Terminator
  transformer1 : powerlib_models/Continuous/hysteresis_transformer  SaturationFlux=SaturationFlux  SaturationCurrent=SaturationCurrent  InitialFlux=InitialFlux1  FluxBase=BaseFlux  CurrentBase=BaseCurrent  Tolerances=Tolerances  HT=HT  UpperFlux=UpperFlux  LowerFlux=LowerFlux  Current=Current  InitialSlope=InitialSlope  TransfoNumber=TransfoNumber1  sfun_InitialFlux=sfun_InitialFlux1
  transformer2 : powerlib_models/Continuous/hysteresis_transformer  SaturationFlux=SaturationFlux  SaturationCurrent=SaturationCurrent  InitialFlux=InitialFlux2  FluxBase=BaseFlux  CurrentBase=BaseCurrent  Tolerances=Tolerances  HT=HT  UpperFlux=UpperFlux  LowerFlux=LowerFlux  Current=Current  InitialSlope=InitialSlope  TransfoNumber=TransfoNumber2  sfun_InitialFlux=sfun_InitialFlux2
  transformer3 : powerlib_models/Continuous/hysteresis_transformer  SaturationFlux=SaturationFlux  SaturationCurrent=SaturationCurrent  InitialFlux=InitialFlux3  FluxBase=BaseFlux  CurrentBase=BaseCurrent  Tolerances=Tolerances  HT=HT  UpperFlux=UpperFlux  LowerFlux=LowerFlux  Current=Current  InitialSlope=InitialSlope  TransfoNumber=TransfoNumber3  sfun_InitialFlux=sfun_InitialFlux3
  tag scope: LibraryTag=global
  wires:
  transformer3/2 -> Goto6/1
  transformer2/2 -> Goto4/1
  transformer1/2 -> Goto2/1
  [LibraryTag] -> transformer1/1
  [LibraryTag] -> transformer2/1
  [LibraryTag] -> transformer3/1
  transformer1/1 -> [LibraryTag]
  transformer2/1 -> [LibraryTag]
  transformer3/1 -> [LibraryTag]

== system powerlib_models/Continuous/Xfohyst3PhF ==
  transformer1 : powerlib_models/Continuous/hysteresis_transformer  SaturationFlux=SaturationFlux  SaturationCurrent=SaturationCurrent  InitialFlux=InitialFlux1  FluxBase=BaseFlux  CurrentBase=BaseCurrent  Tolerances=Tolerances  HT=HT  UpperFlux=UpperFlux  LowerFlux=LowerFlux  Current=Current  InitialSlope=InitialSlope  TransfoNumber=TransfoNumber1  sfun_InitialFlux=sfun_InitialFlux1
  transformer2 : powerlib_models/Continuous/hysteresis_transformer  SaturationFlux=SaturationFlux  SaturationCurrent=SaturationCurrent  InitialFlux=InitialFlux2  FluxBase=BaseFlux  CurrentBase=BaseCurrent  Tolerances=Tolerances  HT=HT  UpperFlux=UpperFlux  LowerFlux=LowerFlux  Current=Current  InitialSlope=InitialSlope  TransfoNumber=TransfoNumber2  sfun_InitialFlux=sfun_InitialFlux2
  transformer3 : powerlib_models/Continuous/hysteresis_transformer  SaturationFlux=SaturationFlux  SaturationCurrent=SaturationCurrent  InitialFlux=InitialFlux3  FluxBase=BaseFlux  CurrentBase=BaseCurrent  Tolerances=Tolerances  HT=HT  UpperFlux=UpperFlux  LowerFlux=LowerFlux  Current=Current  InitialSlope=InitialSlope  TransfoNumber=TransfoNumber3  sfun_InitialFlux=sfun_InitialFlux3
  tag scope: LibraryTag=global
  wires:
  transformer3/2 -> [LibraryTag]
  transformer3/1 -> [LibraryTag]
  transformer2/2 -> [LibraryTag]
  transformer2/1 -> [LibraryTag]
  transformer1/2 -> [LibraryTag]
  transformer1/1 -> [LibraryTag]
  [LibraryTag] -> transformer3/1
  [LibraryTag] -> transformer2/1
  [LibraryTag] -> transformer1/1

== system powerlib_models/Continuous/Xfosat1Ph ==
  Goto2 : Terminator
  transformer : powerlib_models/Continuous/saturable_transformer  SaturationFlux=SaturationFlux  SaturationCurrent=SaturationCurrent  InitialFlux=InitialFlux
  tag scope: LibraryTag=global
  wires:
  transformer/2 -> Goto2/1
  [LibraryTag] -> transformer/1
  transformer/1 -> [LibraryTag]

== system powerlib_models/Continuous/Xfosat1PhF ==
  transformer : powerlib_models/Continuous/saturable_transformer  SaturationFlux=SaturationFlux  SaturationCurrent=SaturationCurrent  InitialFlux=InitialFlux
  tag scope: LibraryTag=global
  wires:
  transformer/2 -> [LibraryTag]
  transformer/1 -> [LibraryTag]
  [LibraryTag] -> transformer/1

== system powerlib_models/Continuous/Xfosat3Ph ==
  Goto2 : Terminator
  Goto4 : Terminator
  Goto6 : Terminator
  transformer1 : powerlib_models/Continuous/saturable_transformer  SaturationFlux=SaturationFlux  SaturationCurrent=SaturationCurrent  InitialFlux=InitialFlux1
  transformer2 : powerlib_models/Continuous/saturable_transformer  SaturationFlux=SaturationFlux  SaturationCurrent=SaturationCurrent  InitialFlux=InitialFlux2
  transformer3 : powerlib_models/Continuous/saturable_transformer  SaturationFlux=SaturationFlux  SaturationCurrent=SaturationCurrent  InitialFlux=InitialFlux3
  tag scope: LibraryTag=global
  wires:
  transformer3/1 -> [LibraryTag]
  transformer2/1 -> [LibraryTag]
  transformer1/1 -> [LibraryTag]
  [LibraryTag] -> transformer3/1
  [LibraryTag] -> transformer2/1
  [LibraryTag] -> transformer1/1
  transformer1/2 -> Goto2/1
  transformer2/2 -> Goto4/1
  transformer3/2 -> Goto6/1

== system powerlib_models/Continuous/Xfosat3PhF ==
  transformer1 : powerlib_models/Continuous/saturable_transformer  SaturationFlux=SaturationFlux  SaturationCurrent=SaturationCurrent  InitialFlux=InitialFlux1
  transformer2 : powerlib_models/Continuous/saturable_transformer  SaturationFlux=SaturationFlux  SaturationCurrent=SaturationCurrent  InitialFlux=InitialFlux2
  transformer3 : powerlib_models/Continuous/saturable_transformer  SaturationFlux=SaturationFlux  SaturationCurrent=SaturationCurrent  InitialFlux=InitialFlux3
  tag scope: LibraryTag=global
  wires:
  [LibraryTag] -> transformer1/1
  [LibraryTag] -> transformer2/1
  [LibraryTag] -> transformer3/1
  transformer1/1 -> [LibraryTag]
  transformer1/2 -> [LibraryTag]
  transformer2/1 -> [LibraryTag]
  transformer2/2 -> [LibraryTag]
  transformer3/1 -> [LibraryTag]
  transformer3/2 -> [LibraryTag]

== system powerlib_models/Continuous/asynchronous_machine ==
  v : Inport  Port=1  LatchInput=off
  thr,wr : Inport  Port=2  LatchInput=off
  Gain : Gain  Gain=[ib2*ones(5,1);phib2;phib2;Vb2;Vb2;ib2*ones(5,1);phib2;phib2;Vb2;Vb2]  SaturateOnIntegerOverflow=on
  Mutual fluxes : Subsystem  Orientation=left
  Mux3 : Mux  Inputs=[3,2,2,2,3,2,2,2]
  Product1 : Product  Inputs=1  SaturateOnIntegerOverflow=on  InputSameDT=on
  Product2 : Product  Inputs=1  SaturateOnIntegerOverflow=on  InputSameDT=on
  Rotor : Subsystem
      mask Display: disp('Rotor')
  Selector : Selector  Elements=[1 4]  InputPortWidth=4
  Selector1 : Selector  Elements=[2 3]  InputPortWidth=4
  Stator : Subsystem
      mask Display: disp('Stator')
  Sum1 : Sum  Inputs=|-+  SaturateOnIntegerOverflow=on  InputSameDT=on
  abc2qd : Subsystem
      mask Display: disp('abc2qd')
  dq2abc : Subsystem
  sin,cos : Subsystem
  i : Outport
  m : Outport  Port=2
  Te : Outport  Port=3
  wires:
  dq2abc/2(irabc) -> Mux3/1
  dq2abc/3(isabc) -> Mux3/5
  Gain/1 -> m/1
  Mux3/1 -> Gain/1
  Stator/2(iqs,ids) -> Mux3/6, dq2abc/3(iqs,ids)
  Stator/1(phiqs,phids) -> Mux3/7, Mutual fluxes/2(phiqs,phids)
  v/1 -> abc2qd/1(v)
  Rotor/1(iqr,idr) -> dq2abc/2(iqr,idr), Mux3/2
  Rotor/2(phiqr,phidr) -> Mux3/3, Mutual fluxes/1(phiqr,phidr)
  dq2abc/1(irab,isab) -> i/1
  abc2qd/1(vqr,vdr) -> Mux3/4, Rotor/1(vqr,vdr)
  abc2qd/2(vqs,vds) -> Mux3/8, Stator/2(vqs,vds)
  sin,cos/3(w) -> Stator/3(w)
  sin,cos/1(sin,cos) -> dq2abc/1(sin,cos), abc2qd/2(sin,cos)
  Mutual fluxes/1(phimq,phimd) -> Stator/1(phimq,phimd), Rotor/3(phimq,phimd)
  sin,cos/2(w-wr) -> Rotor/2(w-wr)
  Stator/3(phis,is) -> Selector/1, Selector1/1
  thr,wr/1 -> sin,cos/1(thr,wr)
  Selector/1 -> Product1/1
  Selector1/1 -> Product2/1
  Product2/1 -> Sum1/2
  Product1/1 -> Sum1/1
  Sum1/1 -> Te/1

== system powerlib_models/Continuous/breaker ==
  v : Inport  Port=1  LatchInput=off
  g : Inport  Port=2  LatchInput=off
  Break Algebraic Loop : Subsystem  mask{Nsw=1, istate=istate}
      mask prompts: Nsw "number of switches"; istate "initial condition"
  Constant : Constant  Value=zeros(Nsw,1)
  S function : S-Function  FunctionName=sfun_psbbreaker  Parameters=istate
  i : Outport  InitialOutput=0
  Status : Outport  Port=2  InitialOutput=0
  wires:
  Constant/1 -> i/1
  v/1 -> S function/1  "Breaker voltage"
  S function/1 -> Break Algebraic Loop/1(In1)  "status"
  g/1 -> S function/2  "gate signal"
  Break Algebraic Loop/1(Out1) -> Status/1

== system powerlib_models/Continuous/detailed_thyristor (logical) ==
  v : Inport  Port=1  LatchInput=off
  g : Inport  Port=2  LatchInput=off
  0 {1..4} (4 alike) : Constant  Value=0
  1/Rsw : Gain  Orientation=down  Gain=1./Rsw  SaturateOnIntegerOverflow=on
  Break Alg. Loop : Subsystem  mask{Nsw=1}
      mask prompts: Nsw "number of switches"
  Constant : Constant  Value=zeros(Nsw,1)
  Data Type  Conversion{1..4} (4 alike) : DataTypeConversion  OutDataTypeMode=boolean  SaturateOnIntegerOverflow=on  RndMeth=Zero
  Mux : Mux  Inputs=2
  Saturation : Saturate  UpperLimit=inf  LowerLimit=0
  Sum : Sum  Inputs=|++  SaturateOnIntegerOverflow=on  InputSameDT=on
  Switch : Switch  Threshold=0.5  InputSameDT=on
  b5 : RelationalOperator  Operator=>  InputSameDT=on
  b6 : RelationalOperator  Operator=>  InputSameDT=on
  b7 : RelationalOperator  Operator===  InputSameDT=on
  or2 : Logic  Operator=OR
  or3 : Logic  Inputs=3
  vf : Constant  Value=Vf
  i : Outport  InitialOutput=0
  Status : Outport  Port=2  InitialOutput=0
  m : Outport  Port=3  InitialOutput=0
  Vf : Outport  Port=4  InitialOutput=0
  wires:
  0 2/1 -> b6/2
  or3/1 -> or2/2  "Fire"
  Mux/1 -> m/1  "measurement signals"
  0 3/1 -> b7/2
  or2/1 -> Break Alg. Loop/1(In1)
  Break Alg. Loop/1(Out1) -> Status/1, Switch/2
  0 1/1 -> b5/2
  Constant/1 -> i/1
  v/1 -> Sum/1, b6/1, 1/Rsw/1  "Vak"
  Sum/1 -> Mux/2
  vf/1 -> Vf/1, Sum/2
  Data Type  Conversion4/1 -> or3/2  "Current = 0"
  b5/1 -> Data Type  Conversion1/1
  Data Type  Conversion1/1 -> or2/1  "Current > 0"
  b6/1 -> Data Type  Conversion2/1
  Data Type  Conversion2/1 -> or3/1  "Voltage > 0"
  Data Type  Conversion3/1 -> or3/3  "Gate = 1"
  b7/1 -> Data Type  Conversion4/1
  g/1 -> Data Type  Conversion3/1
  Switch/1 -> Saturation/1
  0 4/1 -> Switch/3
  Saturation/1 -> Mux/1, b7/1, b5/1
  1/Rsw/1 -> Switch/1  "Iak"
